simulink library "TMotor_F80"  (R2020b)
settings: Solver=VariableStepAuto  StartTime=0.0  StopTime=10.0  RelTol=1e-3
libraries: $bdroot x4
settings Model: Creator=bele  LastModifiedBy=bele

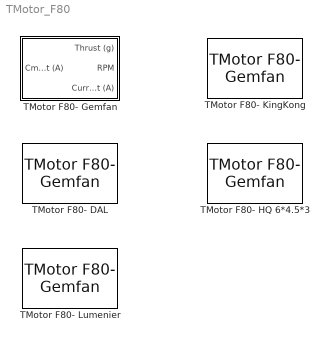
== system TMotor_F80 ==
  TMotor F80- DAL : $bdroot/TMotor F80- Gemfan  SystemSampleTime=-1  VariantActivationTime=update diagram  Latency=0  AutoFrameSizeCalculation=off
      link override Current to RPM: BreakpointsForDimension1=[0 0.99 2.41 7.21 16.49 31.42]  Table=[0 4808 9420 16000 22210 27896]
      link override Current to Thrust: BreakpointsForDimension1=[0 0.99 2.41 7.21 16.49 31.42]  Table=[0 35 144 432 837 1317]
  TMotor F80- Gemfan : Subsystem
  TMotor F80- HQ 6*4.5*3 : $bdroot/TMotor F80- Gemfan  SystemSampleTime=-1  VariantActivationTime=update diagram  Latency=0  AutoFrameSizeCalculation=off
      link override Current to RPM: BreakpointsForDimension1=[0 1.19 3.21 10.29 25.02 48.30]  Table=[0 4669 8915 14611 20047 24343]
      link override Current to Thrust: BreakpointsForDimension1=[0 1.19 3.21 10.29 25.02 48.30]  Table=[0 58 235 661 1242 1910]
  TMotor F80- KingKong : $bdroot/TMotor F80- Gemfan  SystemSampleTime=-1  VariantActivationTime=update diagram  Latency=0  AutoFrameSizeCalculation=off
      link override Current to RPM: BreakpointsForDimension1=[0 1.06 2.52 7.76 18.28 37.24]  Table=[0 4775 9325 15720 21565 26888]
      link override Current to Thrust: BreakpointsForDimension1=[0 1.06 2.52 7.76 18.28 37.24]  Table=[0 39 160 497 1004 1655]
  TMotor F80- Lumenier : $bdroot/TMotor F80- Gemfan  SystemSampleTime=-1  VariantActivationTime=update diagram  Latency=0  AutoFrameSizeCalculation=off
      link override Current to RPM: BreakpointsForDimension1=[0 1.01 2.19 6.40 15.01 30.54]  Table=[0 4853 9528 16272 22603 28249]
      link override Current to Thrust: BreakpointsForDimension1=[0 1.01 2.19 6.40 15.01 30.54]  Table=[0 27 121 388 795 1319]

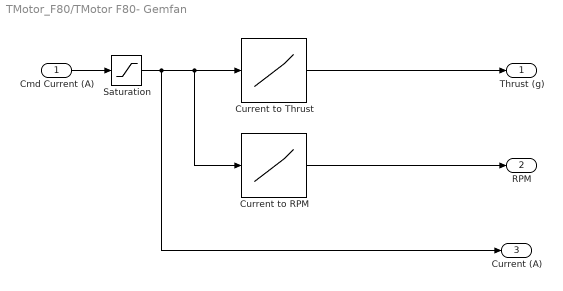
== system TMotor_F80/TMotor F80- Gemfan ==
  Cmd Current (A) : Inport
  Current to RPM : Lookup_n-D  NumberOfTableDimensions=1  BreakpointsForDimension1=[0 1.05 2.50 7.45 16.94 33.24]  Table=[0 4771 9337 15860 21785 27787]  ExtrapMethod=Clip  UseLastTableValue=on  InternalRulePriority=Speed  RndMeth=Simplest  InputSameDT=on
  Current to Thrust : Lookup_n-D  NumberOfTableDimensions=1  BreakpointsForDimension1=[0 1.05 2.50 7.45 16.94 33.24]  Table=[0 37 147 427 816 1310]  ExtrapMethod=Clip  UseLastTableValue=on  InternalRulePriority=Speed  RndMeth=Simplest  InputSameDT=on
  Saturation : Saturate  UpperLimit=33.24  LowerLimit=0
  Thrust (g) : Outport
  RPM : Outport  Port=2
  Current (A) : Outport  Port=3
  wires:
  Cmd Current (A)/1 -> Saturation/1
  Current to RPM/1 -> RPM/1
  Current to Thrust/1 -> Thrust (g)/1
  Saturation/1 -> Current (A)/1, Current to RPM/1, Current to Thrust/1
